simulink model "Kalman_observer"  (R2018b)
settings: Solver=VariableStepAuto  StartTime=0.0  StopTime=10  RelTol=1e-3
InitFcn:
  | % NOTE: If using VoltPAQ-X1, make sure both Gain switches are set to 3.
  | K_AMP = 3;
  | % Maximum Output Voltage (V): YAW limited to 15 V. PITCH limited to 24 V.
  | VMAX_AMP_P = 24;
  | VMAX_AMP_Y = 15;
  | % Initial Angle of Pitch (rad)
  | theta_0 = -40.5*pi/180;
  | 
  | g = 9.81;
  | 
  | % Pitch and Yaw Motor Armature Resistance (Ohm)
  | R_m_p = 0.83;
  | R_m_y = 1.60;
  | 
  | % Pitch and Yaw Motor Current-Torque Constant (N.m/A)
  | K_t_p = 0.0182;
  | K_t_y = 0.0109;
  | 
  | % Pitch and Yaw Motor Voltage-Torque Constant (N.m/V)
  | K_yp = K_t_p / R_m_p;
  | K_py = K_t_y / R_m_y;
  | 
  | % Pitch and Yaw Viscous Damping Constant (N.m.s/rad)
  | B_p = 0.8;  % tuned while running simulation and experiment in parallel
  | B_y = 0.318; % identified as described in manual
  | 
  | % Mass of the Helicopter (kg)
  | m_heli = 1.3872;
  | 
  | % Mass of the Helicopter with Yoke (kg)
  | m_heli_case = 1.421;
  | 
  | % Distance from Pitch Pivot to Pitch/Front Motor and Yaw/Back Motor(m)
  | r_p = 7.75*0.0254;
  | r_y = (6+5/8)*0.0254;
  | 
  | % Pitch and Yaw Propeller Force-Thrust Constant found Experimentally (N/V)
  | K_f_p = 5*0.2074;
  | K_f_y = 3*0.1426;
  | 
  | % Pitch and Yaw Propeller Torque-Thrust Constant found Experimentally (N.m/V)
  | K_pp = K_f_p * r_p;
  | K_yy = K_f_y * r_y;
  | 
  | % Mass of Pitch/Front Motor and Yaw/Back Motor (kg)
  | m_motor_p = 0.292;
  | m_motor_y = 0.128;
  | 
  | % Mass of Pitch/Front and Yaw/Back Guard + Propeller(kg)
  | m_shield = 0.143 + 0.024;
  | 
  | % Total Mass of Pitch and Yaw Motor/Shield Assemblies (kg)
  | m_props = ( m_motor_p + m_motor_y + 2 * m_shield );
  | 
  | % Mass of Helicopter Body moving about Pitch Axis (kg)
  | m_body_p = m_heli - m_props;
  | 
  | % Mass of Helicopter Body moving about Yaw Axis (kg)
  | m_body_y = m_heli_case - m_props;
  | 
  | % Mass of Metal Shaft Moving about Yaw Axis (kg)
  | m_shaft = 0.151;
  | 
  | % Total Length of Helicopter Body (m)
  | L_body = 19*0.0254;
  | 
  | % Helicopter Center of Mass from Pivot along Pitch Axis (m)
  | l_cm = ( (m_motor_p + m_shield ) * r_p +  (m_motor_y + m_shield ) * r_y ) / ( m_props ) ;
  | 
  | % Length of Metal Shaft Moving about Yaw Axis through slip ring (m)
  | L_shaft = 11 * 0.0254;
  | 
  | % Pitch and Yaw Motor Rotor Moment of Inertia (kg.m^2)
  | J_m_p = 1.91e-6; %1.7070e-5;
  | J_m_y = 1.374e-4; %1.4471e-5;
  | 
  | % Moment of Inertia of Helicopter Body about its CM (kg.m^2)
  | J_body_p = m_body_p * L_body^2 / 12;
  | J_body_y = m_body_y * L_body^2 / 12;
  | 
  | % Moment of Inertia of Metal Shaft about Yaw Axis (kg.m^2)
  | J_shaft = m_shaft * L_shaft^2 / 3; %;0.0851;
  | 
  | % Moment of Inertia of Pitch Motor + Guard Assembly about Pivot (kg.m^2)
  | J_p = ( m_motor_p + m_shield ) * r_p^2;
  | 
  | % Moment of Inertia of Yaw Motor + Guard Assembly about Pivot (kg.m^2)
  | J_y = ( m_motor_y + m_shield ) * r_y^2;
  | 
  | % Equivalent Moment of Inertia about Pitch and Yaw Axis (kg.m^2)
  | J_eq_p = J_m_p + J_body_p + J_p + J_y;
  | J_eq_y = J_m_y + J_body_y + J_p + J_y + J_shaft;
  | 
  | 
  | %BESSEL wn=4
  | Kbes=[     68.5119  -25.1203    5.3421   -3.6881
  |    63.1652  188.4894    0.7783   19.4789];
  | 
  | xd=-20;
  | 
  | A=[      0         0    1.0000         0
  |          0         0         0    1.0000
  |          0         0   -9.2751         0
  |          0         0         0   -3.4955];
  | 
  | B=[      0         0
  |          0         0
  |     2.3667    0.0790
  |     0.2410    0.7913];
  | C=eye(4);
  | D = zeros(4,2);
undefined symbols (not defined in the file or in its folder): Continuous, Time
libraries: simulink x1, ctrlSharedLib x1
settings Model: Creator=rezan  LastModifiedBy=rezan
settings DataIOCC: ReturnWorkspaceOutputs=on
settings DebuggingCC: UnconnectedInputMsg=none  UnconnectedOutputMsg=none  UnconnectedLineMsg=none  SFMachineParentedDataDiag=error

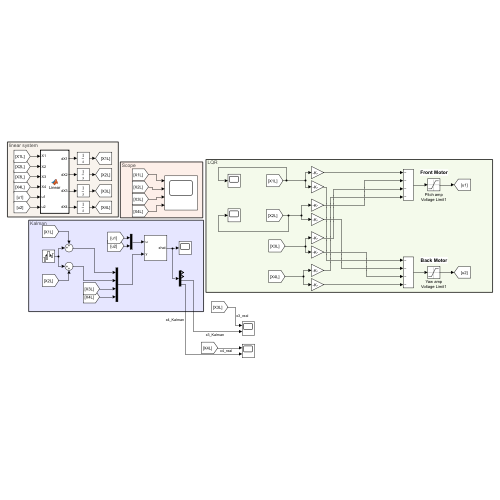
[thumbnail: Simulink's stored preview of the top-level diagram]
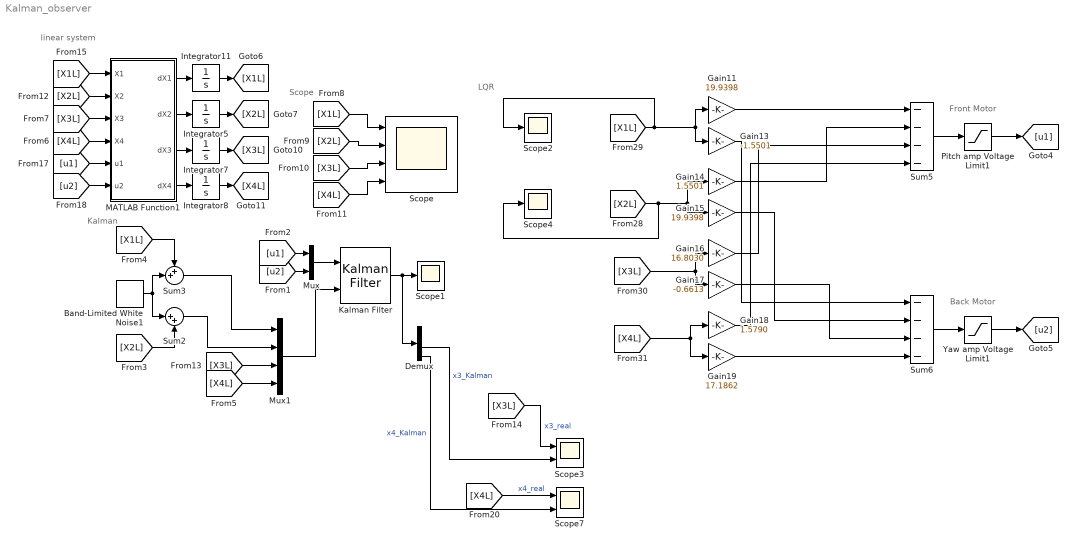
== system Kalman_observer ==
  note: Kalman
  note: linear system
  note: LQR
  note: Scope
  note: Back Motor
  note: Front Motor
  Band-Limited White Noise1 : simulink/Sources/Band-Limited White Noise  Cov=[0.1]  Ts=0.1  seed=[23341]
  Demux : Demux
  Gain11 : Gain  Gain=19.9398
  Gain13 : Gain  Gain=-1.5501
  Gain14 : Gain  Gain=1.5501
  Gain15 : Gain  Gain=19.9398
  Gain16 : Gain  Gain=16.8030
  Gain17 : Gain  Gain=-0.6613
  Gain18 : Gain  Gain=1.5790
  Gain19 : Gain  Gain=17.1862
  Integrator11 : Integrator  UpperSaturationLimit=40.5*pi/180  LowerSaturationLimit=-40.5*pi/180
  Integrator5 : Integrator  InitialCondition=10*pi/180
  Integrator7 : Integrator
  Integrator8 : Integrator
  Kalman Filter : ctrlSharedLib/Kalman Filter  TimeDomain=Continuous-Time  UseCurrentEstimator=on  ModelSource=LTI State-Space Variable  ModelSourceVariable=ss(A,B,C,D)  A=0.95  B=1  C=1  D=0  NumberOfStates=1  NumberOfInputs=1  NumberOfOutputs=1  InitialEstimateSource=Dialog  X0=[0,10*pi/180,0,0]  P0=10  UseK=off  UseGH=off  NumberOfProcessNoiseInputs=1  G=1  TimeInvariantG=on  H=0  TimeInvariantH=on  Q=0.1  TimeInvariantQ=on  R=1  TimeInvariantR=on  N=0  TimeInvariantN=on  AddInputPort=on  AddEnablePort=off  OutputEstimatedY=off  OutputP=off  Ts=-1
  MATLAB Function1 : MATLAB Function  TreatAsAtomicUnit=on
  Mux : Mux  Inputs=2
  Mux1 : Mux
  Pitch amp Voltage Limit1 : Saturate  UpperLimit=VMAX_AMP_P  LowerLimit=- VMAX_AMP_P
  Scope : Scope  NumInputPorts=4
  Scope1 : Scope
  Scope2 : Scope
  Scope3 : Scope  NumInputPorts=2
  Scope4 : Scope
  Scope7 : Scope  NumInputPorts=2
  Sum2 : Sum  Inputs=|++
  Sum3 : Sum  Inputs=++|
  Sum5 : Sum  Inputs=----
  Sum6 : Sum  Inputs=----
  Yaw amp Voltage Limit1 : Saturate  UpperLimit=VMAX_AMP_Y  LowerLimit=- VMAX_AMP_Y
  wires:
  Sum5/1 -> Pitch amp Voltage Limit1/1
  Gain16/1 -> Sum5/3
  [X1L] -> Gain13/1, Gain11/1, Scope2/1
  Gain17/1 -> Sum6/3
  [X2L] -> Gain15/1, Gain14/1, Scope4/1
  Sum6/1 -> Yaw amp Voltage Limit1/1
  Gain13/1 -> Sum6/1
  [X4L] -> Scope/4
  [X2L] -> Scope/2
  Integrator7/1 -> [X3L]
  Gain18/1 -> Sum5/4
  [X3L] -> Gain17/1, Gain16/1
  [X4L] -> MATLAB Function1/4(X4)
  MATLAB Function1/4(dX4) -> Integrator8/1
  Integrator8/1 -> [X4L]
  Gain11/1 -> Sum5/1
  MATLAB Function1/2(dX2) -> Integrator5/1
  Integrator11/1 -> [X1L]
  [X1L] -> Scope/1
  [X3L] -> Scope/3
  MATLAB Function1/1(dX1) -> Integrator11/1
  MATLAB Function1/3(dX3) -> Integrator7/1
  Integrator5/1 -> [X2L]
  [u2] -> MATLAB Function1/6(u2)
  [X4L] -> Gain19/1, Gain18/1
  [X2L] -> MATLAB Function1/2(X2)
  Gain19/1 -> Sum6/4
  [X3L] -> MATLAB Function1/3(X3)
  Gain15/1 -> Sum6/2
  Gain14/1 -> Sum5/2
  [X1L] -> MATLAB Function1/1(X1)
  [u1] -> MATLAB Function1/5(u1)
  Mux/1 -> Kalman Filter/1
  [u1] -> Mux/1
  [u2] -> Mux/2
  Mux1/1 -> Kalman Filter/2
  Band-Limited White Noise1/1 -> Sum3/2, Sum2/1
  [X4L] -> Mux1/4
  [X3L] -> Mux1/3
  [X2L] -> Sum2/2
  [X1L] -> Sum3/1
  Sum3/1 -> Mux1/1
  Sum2/1 -> Mux1/2
  Pitch amp Voltage Limit1/1 -> [u1]
  Yaw amp Voltage Limit1/1 -> [u2]
  Kalman Filter/1 -> Demux/1, Scope1/1
  [X3L] -> Scope3/1  "x3_real"
  Demux/3 -> Scope3/2  "x3_Kalman"
  [X4L] -> Scope7/1  "x4_real"
  Demux/4 -> Scope7/2  "x4_Kalman"

== matlab function Kalman_observer/MATLAB Function1 ==
  data: X1 input; dX1 output; X2 input; X3 input; X4 input; u1 input; dX2 output; dX3 output; dX4 output; u2 input
function [dX1,dX2,dX3,dX4] = Linear(X1,X2,X3,X4,u1,u2)
%#codegen

A=[      0         0    1.0000         0
         0         0         0    1.0000
         0         0   -9.2751         0
         0         0         0   -3.4955];
     
B=[      0         0
         0         0
    2.3667    0.0790
    0.2410    0.7913];

X = [X1;X2;X3;X4];
U=[u1,u2].';
dX = A*X+B*U;
dX1 = dX(1);
dX2 = dX(2);
dX3 = dX(3);
dX4 = dX(4);
